simulink model "ship4dof"  (R2019b)
settings: Solver=ode4  StartTime=0.0  StopTime=tEnd  FixedStep=tStep  RelTol=1e-3
values from neighbouring files (symbols this model uses):
  AOA = block.InputPort(1).Data    [force_wing.m]
  W_theta = wind_vector(2)    [force_wing.m]
  Wv = wind_vector(1)    [force_wing.m]
undefined symbols (not defined in the file or in its folder): delta, ics, kd_t, kd_u, ki_t, ki_u, kp_t, kp_u, lim, ship, Thrust, u_d, z_d
libraries: simulink x2
settings Model: Creator=e_anderlini  LastModifiedBy=arthu
settings SFSimCC: CustomCodeUndefinedFunction=UseInterfaceOnly

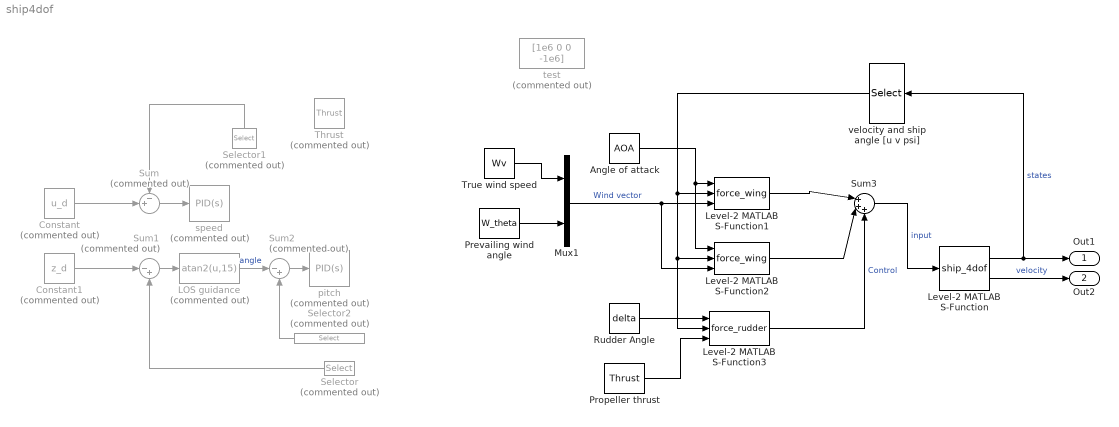
== system ship4dof ==
  Angle of attack : Constant  Value=AOA
  Constant : Constant  Commented=on  Value=u_d
  Constant1 : Constant  Commented=on  Value=z_d
  LOS guidance : Fcn  Commented=on  Expr=atan2(u,15)
  Level-2 MATLAB S-Function : M-S-Function  FunctionName=ship_4dof  Parameters=ship.propulsion,ship.actuators,ship.rigid_body,ship.X,ship.Y,ship.N,ship.K,ship.Minv,ics
  Level-2 MATLAB S-Function1 : M-S-Function  FunctionName=force_wing  Parameters=ship.wing,ship.d_bow,ship.Cl_angle,ship.Cl_data,ship.Cd_angle,ship.Cd_data,ship.wind_oriantation,ship.Cl_ratio_bow,ship.Cd_ratio_bow
  Level-2 MATLAB S-Function2 : M-S-Function  FunctionName=force_wing  Parameters=ship.wing,ship.d_stern,ship.Cl_angle,ship.Cl_data,ship.Cd_angle,ship.Cd_data,ship.wind_oriantation,ship.Cl_ratio_stern,ship.Cd_ratio_stern
  Level-2 MATLAB S-Function3 : M-S-Function  FunctionName=force_rudder  Parameters=ship.rud,ship.d_rud,ship.AOA_rud,ship.Cl_rud,ship.Cd_rud
  Mux1 : Mux  Inputs=2
  Prevailing wind angle : Constant  Value=W_theta
  Propeller thrust : Constant  Value=Thrust
  Rudder Angle : Constant  Value=delta
  Selector : Selector  Commented=on  InputPortWidth=10  IndexOptions=Index vector (dialog)  Indices=[2]  OutputSizes=1
  Selector1 : Selector  Commented=on  InputPortWidth=10  IndexOptions=Index vector (dialog)  Indices=[4]  OutputSizes=1
  Selector2 : Selector  Commented=on  InputPortWidth=10  IndexOptions=Index vector (dialog)  Indices=[3]  OutputSizes=1
  Sum : Sum  Commented=on  Inputs=-+|
  Sum1 : Sum  Commented=on  Inputs=|-+
  Sum2 : Sum  Commented=on  Inputs=|-+
  Sum3 : Sum  Inputs=|+++
  Thrust : Constant  Commented=on  Value=Thrust
  True wind speed : Constant  Value=Wv
  pitch : simulink/Continuous/PID Controller  Commented=on  Controller=PID  Form=Parallel  TimeDomain=Continuous-time  SampleTime=-1  IntegratorMethod=Forward Euler  FilterMethod=Forward Euler  ControllerParametersSource=internal  P=kp_t  I=ki_t  D=kd_t  UseFilter=on  N=100  TunerSelectOption=Transfer Function Based (PID Tuner App)  InitialConditionSource=internal  InitialConditionForIntegrator=0  InitialConditionForFilter=0  DifferentiatorICPrevScaledInput=0  ExternalReset=none  TrackingMode=off  Kt=1  LimitOutput=on  UpperSaturationLimit=lim.angle  LowerSaturationLimit=-lim.angle  LinearizeAsGain=on  AntiWindupMode=none  Kb=1  POutMin=[]  POutMax=[]  IOutMin=[]  IOutMax=[]  DOutMin=[]  DOutMax=[]  NOutMin=[]  NOutMax=[]  SumOutMin=[]  SumOutMax=[]  SaturationOutMin=[]  SaturationOutMax=[]  PParamMin=[]  PParamMax=[]  IParamMin=[]  IParamMax=[]  DParamMin=[]  DParamMax=[]  NParamMin=[]  NParamMax=[]  KbParamMin=[]  KbParamMax=[]  KtParamMin=[]  KtParamMax=[]  KbOutMin=[]  KbOutMax=[]  KtOutMin=[]  KtOutMax=[]  IntegratorOutMin=[]  IntegratorOutMax=[]  FilterOutMin=[]  FilterOutMax=[]  SumI1OutMin=[]  SumI1OutMax=[]  SumI2OutMin=[]  SumI2OutMax=[]  SumI3OutMin=[]  SumI3OutMax=[]  SumI4OutMin=[]  SumI4OutMax=[]  SumDOutMin=[]  SumDOutMax=[]  DifferentiatorOutMin=[]  DifferentiatorOutMax=[]  FilterDiffOutCoefMin=[]  FilterDiffOutCoefMax=[]  ReciprocalOutMin=[]  ReciprocalOutMax=[]  SumDenOutMin=[]  SumDenOutMax=[]  SumNumOutMin=[]  SumNumOutMax=[]  DivideOutMin=[]  DivideOutMax=[]  IntegratorContinuousStateAttributes=''  IntegratorStateMustResolveToSignalObject=off  IntegratorRTWStateStorageClass=Auto  FilterContinuousStateAttributes=''  FilterStateMustResolveToSignalObject=off  FilterRTWStateStorageClass=Auto  ParallelPVariant=InternalParameters  IdealPVariant=Disabled  IVariant=InternalParameters  DVariant=InternalParameters  IntegratorVariant=Continuous  SatVariant=Enabled  AWVariant=Passthrough  PCopyVariant=Disabled  TRVariant=Disabled  FdbkBlocksVariant=Forward  IdealPFdbkVariant=Disabled  SatFdbkVariant=Disabled  DerivativeFilterVariant=ContFilter  NVariant=InternalParameters  NCopyVariant=Disabled  FilterICVariant=InternalICsFilter  IntegratorICVariant=InternalICs  ExternalResetVariant=Disabled  TRSumVariant=Passthrough  SumFdbkVariant=Disabled  SumVariant=Sum_PID
  speed : simulink/Continuous/PID Controller  Commented=on  Controller=PID  Form=Parallel  TimeDomain=Continuous-time  SampleTime=-1  IntegratorMethod=Forward Euler  FilterMethod=Forward Euler  ControllerParametersSource=internal  P=kp_u  I=ki_u  D=kd_u  UseFilter=on  N=100  TunerSelectOption=Transfer Function Based (PID Tuner App)  InitialConditionSource=internal  InitialConditionForIntegrator=0  InitialConditionForFilter=0  DifferentiatorICPrevScaledInput=0  ExternalReset=none  TrackingMode=off  Kt=1  LimitOutput=on  UpperSaturationLimit=lim.torque  LowerSaturationLimit=-lim.torque  LinearizeAsGain=on  AntiWindupMode=none  Kb=1  POutMin=[]  POutMax=[]  IOutMin=[]  IOutMax=[]  DOutMin=[]  DOutMax=[]  NOutMin=[]  NOutMax=[]  SumOutMin=[]  SumOutMax=[]  SaturationOutMin=[]  SaturationOutMax=[]  PParamMin=[]  PParamMax=[]  IParamMin=[]  IParamMax=[]  DParamMin=[]  DParamMax=[]  NParamMin=[]  NParamMax=[]  KbParamMin=[]  KbParamMax=[]  KtParamMin=[]  KtParamMax=[]  KbOutMin=[]  KbOutMax=[]  KtOutMin=[]  KtOutMax=[]  IntegratorOutMin=[]  IntegratorOutMax=[]  FilterOutMin=[]  FilterOutMax=[]  SumI1OutMin=[]  SumI1OutMax=[]  SumI2OutMin=[]  SumI2OutMax=[]  SumI3OutMin=[]  SumI3OutMax=[]  SumI4OutMin=[]  SumI4OutMax=[]  SumDOutMin=[]  SumDOutMax=[]  DifferentiatorOutMin=[]  DifferentiatorOutMax=[]  FilterDiffOutCoefMin=[]  FilterDiffOutCoefMax=[]  ReciprocalOutMin=[]  ReciprocalOutMax=[]  SumDenOutMin=[]  SumDenOutMax=[]  SumNumOutMin=[]  SumNumOutMax=[]  DivideOutMin=[]  DivideOutMax=[]  IntegratorContinuousStateAttributes=''  IntegratorStateMustResolveToSignalObject=off  IntegratorRTWStateStorageClass=Auto  FilterContinuousStateAttributes=''  FilterStateMustResolveToSignalObject=off  FilterRTWStateStorageClass=Auto  ParallelPVariant=InternalParameters  IdealPVariant=Disabled  IVariant=InternalParameters  DVariant=InternalParameters  IntegratorVariant=Continuous  SatVariant=Enabled  AWVariant=Passthrough  PCopyVariant=Disabled  TRVariant=Disabled  FdbkBlocksVariant=Forward  IdealPFdbkVariant=Disabled  SatFdbkVariant=Disabled  DerivativeFilterVariant=ContFilter  NVariant=InternalParameters  NCopyVariant=Disabled  FilterICVariant=InternalICsFilter  IntegratorICVariant=InternalICs  ExternalResetVariant=Disabled  TRSumVariant=Passthrough  SumFdbkVariant=Disabled  SumVariant=Sum_PID
  test : Constant  Commented=on  Value=[1e6 0 0 -1e6]
  velocity and ship angle [u v psi] : Selector  InputPortWidth=8  IndexOptions=Index vector (dialog)  Indices=[5,6,4]  OutputSizes=1
  Out1 : Outport  VectorParamsAs1DForOutWhenUnconnected=off
  Out2 : Outport  Port=2  VectorParamsAs1DForOutWhenUnconnected=off
  wires:
  Selector/1 -> Sum1/2
  Sum/1 -> speed/1
  Constant/1 -> Sum/2
  Constant1/1 -> Sum1/1
  Selector1/1 -> Sum/1
  Level-2 MATLAB S-Function/2 -> Out2/1  "velocity"
  Sum2/1 -> pitch/1
  Selector2/1 -> Sum2/2
  LOS guidance/1 -> Sum2/1  "angle"
  Sum1/1 -> LOS guidance/1
  Rudder Angle/1 -> Level-2 MATLAB S-Function3/1
  True wind speed/1 -> Mux1/1
  Prevailing wind angle/1 -> Mux1/2
  Mux1/1 -> Level-2 MATLAB S-Function1/3, Level-2 MATLAB S-Function2/3  "Wind vector"
  Level-2 MATLAB S-Function2/1 -> Sum3/2
  Angle of attack/1 -> Level-2 MATLAB S-Function1/1, Level-2 MATLAB S-Function2/1
  Level-2 MATLAB S-Function/1 -> Out1/1, velocity and ship angle [u v psi]/1  "states"
  velocity and ship angle [u v psi]/1 -> Level-2 MATLAB S-Function1/2, Level-2 MATLAB S-Function3/2, Level-2 MATLAB S-Function2/2
  Level-2 MATLAB S-Function1/1 -> Sum3/1
  Propeller thrust/1 -> Level-2 MATLAB S-Function3/3
  Sum3/1 -> Level-2 MATLAB S-Function/1  "input"
  Level-2 MATLAB S-Function3/1 -> Sum3/3  "Control"
